simulink model "sim13"  (R2015b)
settings: Solver=VariableStepAuto  StartTime=0.0  StopTime=10.0  RelTol=1e-3
values from neighbouring files (symbols this model uses):
  G = 1/(k-g*(m*l+(1/2)*M*L))    (= 20.7182082927)    [Lab3.m]
  w_teste = w_teste_set(i)    [Lab3.m]
  wn = sqrt((k-g*(m*l+(1/2)*M*L))/J)    [Lab3.m]
  zeta = beta/(2*J*wn)    [Lab3.m]
settings Model: Creator=Alice  LastModifiedBy=Alice

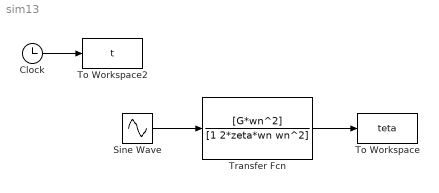
== system sim13 ==
  Clock : Clock
  Sine Wave : Sin  Frequency=w_teste  SampleTime=0
  To Workspace : ToWorkspace  VariableName=teta  SampleTime=0.01
  To Workspace2 : ToWorkspace  VariableName=t  SampleTime=0.01
  Transfer Fcn : TransferFcn  Numerator=[G*wn^2]  Denominator=[1 2*zeta*wn wn^2]
  wires:
  Sine Wave/1 -> Transfer Fcn/1
  Transfer Fcn/1 -> To Workspace/1
  Clock/1 -> To Workspace2/1
